simulink model "speed_current_mech"  (R2024a)
settings: Solver=VariableStepAuto  StartTime=0.0  StopTime=Stop_Time  RelTol=1e-3
values from neighbouring files (symbols this model uses):
  B = 0.001    [main.m]
  Ia_rated = 30    [main.m]
  J = 0.003    [main.m]
  Kac = 1/Kpc    (= 1.59154943092)    [main.m]
  Ke = Kt    (= 0.318309886184)    [main.m]
  Kic = Ra * Wcc    (= 94.2477796077)    [main.m]
  Kis = J*Wsc^2/(5*Kt)    (= 7.44150640327)    [main.m]
  Kpc = La * Wcc    (= 0.628318530718)    [main.m]
  Kps = J*Wsc/Kt    (= 0.592176264065)    [main.m]
  Kt = Te_rated/Ia_rated    (= 0.318309886184)    [main.m]
  La = 2.0e-3    (= 0.002)    [main.m]
  Ra = 0.3    [main.m]
  Va_rated = 100    [main.m]
settings Model: Creator=moon  LastModifiedBy=moon

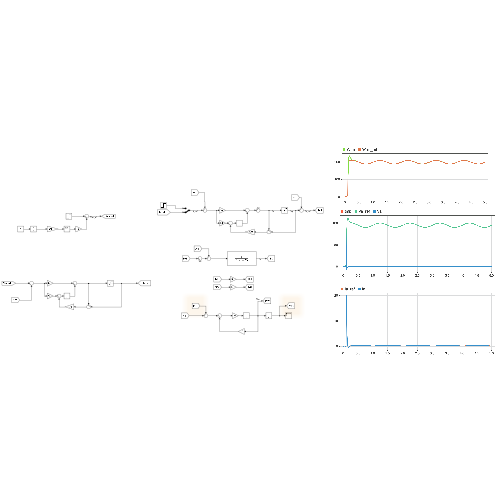
[thumbnail: Simulink's stored preview of the top-level diagram]
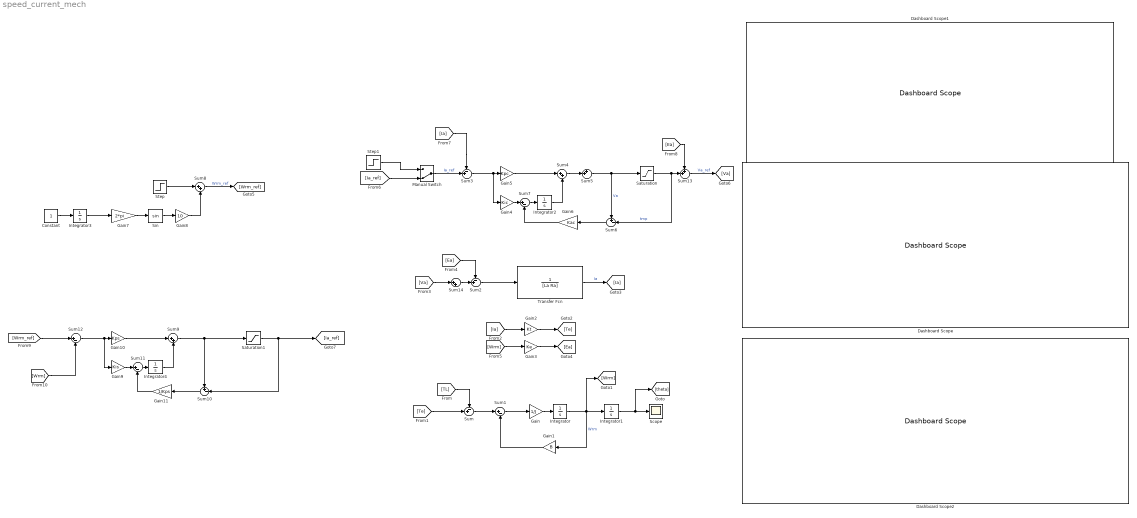
== system speed_current_mech ==
  Constant : Constant
  Dashboard Scope : DashboardScope
  Dashboard Scope1 : DashboardScope
  Dashboard Scope2 : DashboardScope
  Gain : Gain  Gain=1/J
  Gain1 : Gain  Gain=B
  Gain10 : Gain  Gain=Kps
  Gain11 : Gain  Gain=1/Kps
  Gain2 : Gain  Gain=Kt
  Gain3 : Gain  Gain=Ke
  Gain4 : Gain  Gain=Kic
  Gain5 : Gain  Gain=Kpc
  Gain6 : Gain  Gain=Kac
  Gain7 : Gain  Gain=2*pi
  Gain8 : Gain  Gain=10
  Gain9 : Gain  Gain=Kis
  Integrator{,1..4} (5 alike) : Integrator
  Manual Switch : ManualSwitch  CurrentSetting=0
  Saturation : Saturate  UpperLimit=Va_rated  LowerLimit=-Va_rated
  Saturation1 : Saturate  UpperLimit=Ia_rated  LowerLimit=-Ia_rated
  Scope : Scope
  Sin : Trigonometry
  Step : Step  Time=0.1  After=200  SampleTime=0
  Step1 : Step  After=Ia_rated  SampleTime=0
  Sum : Sum  Inputs=-+|
  Sum{1,7,11..12} (4 alike) : Sum  Inputs=|+-
  Sum10 : Sum  Inputs=+-|
  Sum13 : Sum  Inputs=++|
  Sum{4,8..9,14} (4 alike) : Sum  Inputs=|++
  Sum2 : Sum  Inputs=-+|
  Sum3 : Sum  Inputs=-+|
  Sum5 : Sum  Inputs=++|
  Sum6 : Sum  Inputs=+-|
  Transfer Fcn : TransferFcn  Denominator=[La Ra]
  wires:
  [Te] -> Sum/2
  [TL] -> Sum/1
  Sum/1 -> Sum1/1
  Sum1/1 -> Gain/1
  Gain/1 -> Integrator/1
  Gain1/1 -> Sum1/2
  Integrator/1 -> [Wrm], Integrator1/1, Gain1/1  "Wrm"
  Integrator1/1 -> [theta], Scope/1
  [Ia] -> Gain2/1
  Gain2/1 -> [Te]
  Transfer Fcn/1 -> [Ia]  "Ia"
  Sum14/1 -> Sum2/2
  Sum2/1 -> Transfer Fcn/1
  [Ea] -> Sum2/1
  Gain3/1 -> [Ea]
  [Wrm] -> Gain3/1
  Manual Switch/1 -> Sum3/2  "Ia_ref"
  [Ia] -> Sum3/1
  Sum3/1 -> Gain5/1, Gain4/1
  Sum4/1 -> Sum5/2
  Sum5/1 -> Sum6/1, Saturation/1  "Va"
  Saturation/1 -> Sum13/2, Sum6/2  "tmp"
  Sum6/1 -> Gain6/1
  Integrator2/1 -> Sum4/2
  Gain5/1 -> Sum4/1
  Gain4/1 -> Sum7/1
  Sum7/1 -> Integrator2/1
  Gain6/1 -> Sum7/2
  Step/1 -> Sum8/1
  Constant/1 -> Integrator3/1
  Integrator3/1 -> Gain7/1
  Gain7/1 -> Sin/1
  Sin/1 -> Gain8/1
  Gain8/1 -> Sum8/2
  Sum8/1 -> [Wrm_ref]  "Wrm_ref"
  Sum12/1 -> Gain9/1, Gain10/1
  Integrator4/1 -> Sum9/2
  Gain10/1 -> Sum9/1
  Sum9/1 -> Saturation1/1, Sum10/1
  Step1/1 -> Manual Switch/1
  [Ia_ref] -> Manual Switch/2
  Sum10/1 -> Gain11/1
  Gain9/1 -> Sum11/1
  Sum11/1 -> Integrator4/1
  Gain11/1 -> Sum11/2
  Saturation1/1 -> Sum10/2, [Ia_ref]
  [Wrm] -> Sum12/2
  [Wrm_ref] -> Sum12/1
  [Ea] -> Sum13/1
  Sum13/1 -> [Va]  "Va_ref"
  [Va] -> Sum14/1
